simulink model "depth_system"  (R2016b)
settings: Solver=ode45  StartTime=0.0  StopTime=180  RelTol=1e-3  EnableMultiTasking=on
values from neighbouring files (symbols this model uses):
  controllers = pidtune(plants,'p',.1)    [depth_ctl_design.m]
  Fmax = 64    [depth_ctl_design.m]
  G = 9.8    [depth_ctl_design.m]
  Kd = .5*rho*Cd*A    (= 600)    [depth_ctl_design.m]
  M = 45    [depth_ctl_design.m]
  opPoints = linspace(0,Vmax,5)    [depth_ctl_design.m]
  outputDeadZone = 0.1*4    (= 0.4)    [depth_ctl_design.m]
  rho = 1000    [depth_ctl_design.m]
  sensorPeriod = 1/100    (= 0.01)    [depth_ctl_design.m]
  V = .045    (= 0.045)    [depth_ctl_design.m]
undefined symbols (not defined in the file or in its folder): maxF
libraries: simulink x3
settings Model: Creator=Cassandra  LastModifiedBy=Cassandra
settings DataIOCC: LimitDataPoints=on  SaveFormat=Array
settings OptimizationCC: LifeSpan=inf
settings DebuggingCC: MaxConsecutiveZCsMsg=none  SFUnexpectedBacktrackingDiag=warning  SFNoUnconditionalDefaultTransitionDiag=warning  SFExecutionAtInitializationDiag=none
settings HardwareCC: ProdBitPerPointer=32  ProdBitPerSizeT=32  ProdBitPerPtrDiffT=32  ProdLargestAtomicFloat=None  ProdIntDivRoundTo=Undefined  ProdEndianess=Unspecified  ProdWordSize=32  ProdHWDeviceType=32-bit Generic
settings ModelReferenceCC: PropagateSignalLabelsOutOfModel=off
settings GRTTargetCC: TargetLangStandard=C89/C90 (ANSI)  GeneratePreprocessorConditionals=Disable all
settings ConfigComp: CovMetricSettings=dw  CovHtmlReporting=on  CovSaveCumulativeToWorkspaceVar=on  CovSaveSingleToWorkspaceVar=on  CovExternalEMLEnable=off

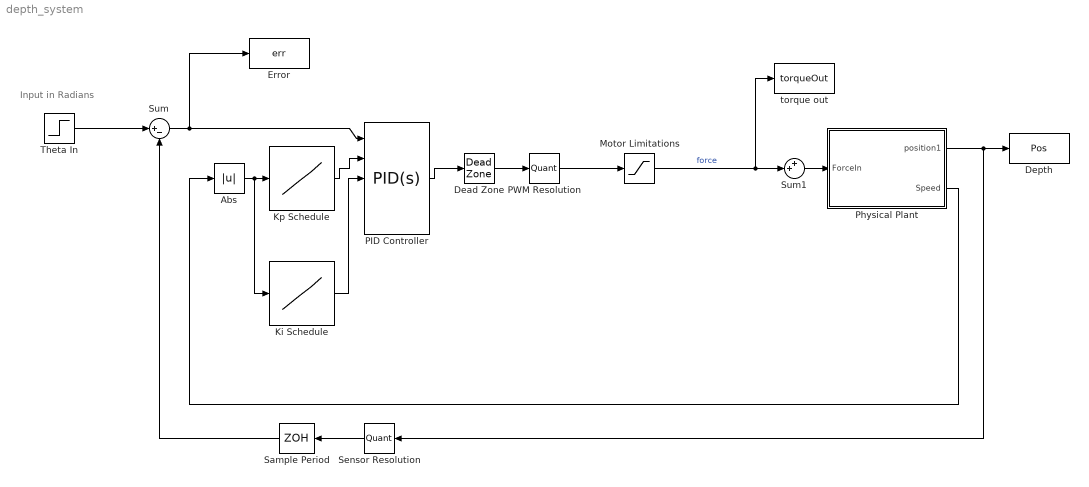
== system depth_system ==
  note: Input in Radians
  Abs : Abs
  Dead Zone : DeadZone  LowerValue=-outputDeadZone  UpperValue=outputDeadZone  SaturateOnIntegerOverflow=on
  Depth : ToWorkspace  VariableName=Pos  SaveFormat=Timeseries  SampleTime=-1
  Error : ToWorkspace  VariableName=err  SaveFormat=Timeseries  SampleTime=-1
  Ki Schedule : Lookup_n-D  NumberOfTableDimensions=1  BreakpointsForDimension1=opPoints  BeginIndexSearchUsingPreviousIndexResult=on  Table=controllers.Ki  UseLastTableValue=on  InternalRulePriority=Speed  RndMeth=Simplest  InputSameDT=on
  Kp Schedule : Lookup_n-D  NumberOfTableDimensions=1  BreakpointsForDimension1=opPoints  BeginIndexSearchUsingPreviousIndexResult=on  Table=controllers.Kp  UseLastTableValue=on  InternalRulePriority=Speed  RndMeth=Simplest  InputSameDT=on
  Motor Limitations : Saturate  UpperLimit=Fmax  LowerLimit=-Fmax
  PID Controller : simulink/Continuous/PID Controller  Controller=PID  TimeDomain=Continuous-time  SampleTime=-1  IntegratorMethod=Forward Euler  FilterMethod=Forward Euler  Form=Parallel  UseFilter=on  ControllerParametersSource=external  P=3608.50201363865  I=36878.829243752  D=54.7457908705096  N=123.498031734756  InitialConditionSource=internal  InitialConditionForIntegrator=0  InitialConditionForFilter=0  ExternalReset=none  LimitOutput=off  UpperSaturationLimit=maxF  LowerSaturationLimit=-maxF  LinearizeAsGain=on  AntiWindupMode=clamping  Kb=1  TrackingMode=off  Kt=1  PParamMin=[]  PParamMax=[]  IParamMin=[]  IParamMax=[]  DParamMin=[]  DParamMax=[]  NParamMin=[]  NParamMax=[]  KbParamMin=[]  KbParamMax=[]  KtParamMin=[]  KtParamMax=[]  POutMin=[]  POutMax=[]  IOutMin=[]  IOutMax=[]  DOutMin=[]  DOutMax=[]  NOutMin=[]  NOutMax=[]  KbOutMin=[]  KbOutMax=[]  KtOutMin=[]  KtOutMax=[]  IntegratorOutMin=[]  IntegratorOutMax=[]  FilterOutMin=[]  FilterOutMax=[]  SumOutMin=[]  SumOutMax=[]  SumI1OutMin=[]  SumI1OutMax=[]  SumI2OutMin=[]  SumI2OutMax=[]  SumI3OutMin=[]  SumI3OutMax=[]  SumDOutMin=[]  SumDOutMax=[]  SaturationOutMin=[]  SaturationOutMax=[]  IntegratorContinuousStateAttributes=''  IntegratorStateMustResolveToSignalObject=off  IntegratorRTWStateStorageClass=Auto  FilterContinuousStateAttributes=''  FilterStateMustResolveToSignalObject=off  FilterRTWStateStorageClass=Auto  DifferentiatorICPrevScaledInput=0  DifferentiatorOutMin=[]  DifferentiatorOutMax=[]
  PWM Resolution : Quantizer  QuantizationInterval=outputResolution
  Physical Plant : Subsystem
  Sample Period : ZeroOrderHold  SampleTime=sensorPeriod
  Sensor Resolution : Quantizer  QuantizationInterval=sensorResolution
  Sum : Sum  Inputs=|+-
  Sum1 : Sum  Inputs=++|
  Theta In : Step  After=2  SampleTime=0
  torque out : ToWorkspace  VariableName=torqueOut  SaveFormat=Timeseries  SampleTime=-1
  wires:
  Theta In/1 -> Sum/1
  PWM Resolution/1 -> Motor Limitations/1
  Sensor Resolution/1 -> Sample Period/1
  PID Controller/1 -> Dead Zone/1
  Abs/1 -> Ki Schedule/1, Kp Schedule/1
  Sum/1 -> PID Controller/1, Error/1
  Sample Period/1 -> Sum/2
  Motor Limitations/1 -> torque out/1, Sum1/2  "force"
  Kp Schedule/1 -> PID Controller/2
  Dead Zone/1 -> PWM Resolution/1
  Physical Plant/1(position1) -> Sensor Resolution/1, Depth/1
  Physical Plant/2(Speed) -> Abs/1
  Sum1/1 -> Physical Plant/1(ForceIn)
  Ki Schedule/1 -> PID Controller/3

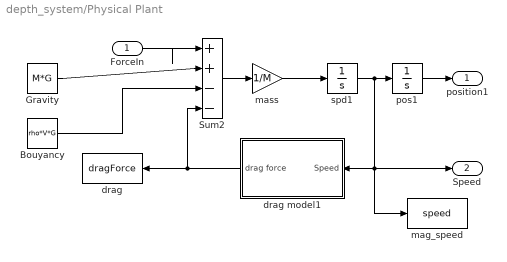
== system depth_system/Physical Plant ==
  ForceIn : Inport
  Bouyancy : Constant  Value=rho*V*G
  Gravity : Constant  Value=M*G
  Sum2 : Sum  Inputs=|++--
  drag : ToWorkspace  VariableName=dragForce  SaveFormat=Timeseries  SampleTime=-1
  drag model1 : Subsystem
  mag_speed : ToWorkspace  VariableName=speed  SaveFormat=Timeseries  SampleTime=-1
  mass : Gain  Gain=1/M
  pos1 : Integrator
  spd1 : Integrator
  position1 : Outport
  Speed : Outport  Port=2
  wires:
  mass/1 -> spd1/1
  spd1/1 -> pos1/1, Speed/1, mag_speed/1, drag model1/1(Speed)
  Sum2/1 -> mass/1
  ForceIn/1 -> Sum2/1
  pos1/1 -> position1/1
  drag model1/1(drag force) -> drag/1, Sum2/4
  Gravity/1 -> Sum2/2
  Bouyancy/1 -> Sum2/3

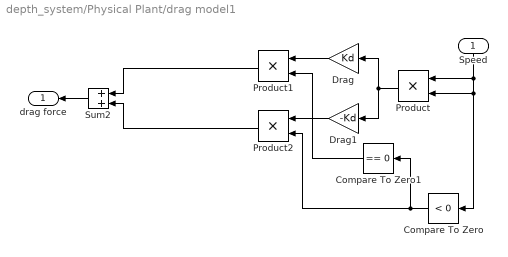
== system depth_system/Physical Plant/drag model1 ==
  Speed : Inport
  Compare To Zero : simulink/Logic and Bit Operations/Compare To Zero  relop=<  OutDataTypeStr=boolean
  Compare To Zero1 : simulink/Logic and Bit Operations/Compare To Zero  relop===  OutDataTypeStr=boolean
  Drag : Gain  Gain=Kd
  Drag1 : Gain  Gain=-Kd
  Product : Product
  Product1 : Product
  Product2 : Product
  Sum2 : Sum  Inputs=+|+
  drag force : Outport
  wires:
  Speed/1 -> Product/1, Compare To Zero/1, Product/2
  Drag1/1 -> Product2/1
  Compare To Zero1/1 -> Product1/2
  Product1/1 -> Sum2/1
  Drag/1 -> Product1/1
  Sum2/1 -> drag force/1
  Product/1 -> Drag1/1, Drag/1
  Product2/1 -> Sum2/2
  Compare To Zero/1 -> Product2/2, Compare To Zero1/1
